simulink model "Dead_Zone_Limit"  (R2012b)
settings: Solver=ode45  StartTime=0.0  StopTime=10.0  RelTol=1e-3
libraries: simulink x1
settings Model: Creator=Faradars  LastModifiedBy=Faradars

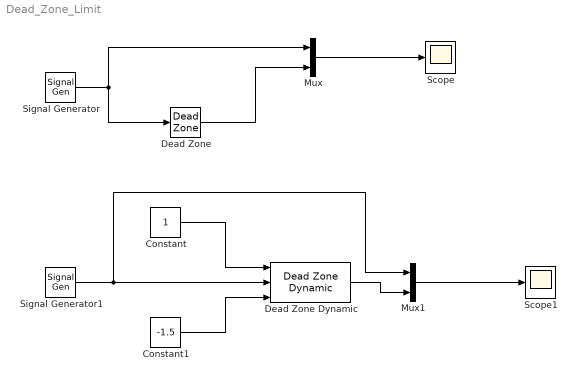
== system Dead_Zone_Limit ==
  Constant : Constant
  Constant1 : Constant  Value=-1.5
  Dead Zone : DeadZone  LowerValue=-0.25  UpperValue=0.25  SaturateOnIntegerOverflow=on
  Dead Zone Dynamic : simulink/Discontinuities/Dead Zone Dynamic
  Mux : Mux  Inputs=2
  Mux1 : Mux  Inputs=2
  Scope : Scope
  Scope1 : Scope
  Signal Generator : SignalGenerator  Frequency=0.2
  Signal Generator1 : SignalGenerator  Amplitude=2  Frequency=0.2
  wires:
  Mux/1 -> Scope/1
  Dead Zone/1 -> Mux/2
  Signal Generator/1 -> Mux/1, Dead Zone/1
  Constant/1 -> Dead Zone Dynamic/1
  Constant1/1 -> Dead Zone Dynamic/3
  Signal Generator1/1 -> Mux1/1, Dead Zone Dynamic/2
  Mux1/1 -> Scope1/1
  Dead Zone Dynamic/1 -> Mux1/2
